simulink model "Calculate_Average_Switching_Frequency"  (R2018a)
settings: Solver=FixedStepAuto  StartTime=0.0  StopTime=0.17  RelTol=1e-3
values from neighbouring files (symbols this model uses):
  f_f_cf = 100e3    (= 100000)    [Init_Average_Switching_Frequency.m]
  f_T_cf = 1/f_f_cf    (= 1e-05)    [Init_Average_Switching_Frequency.m]
  f_T_fpga = 1/f_fpga    (= 1e-08)    [Init_Average_Switching_Frequency.m]
  T_fpga = 1/f_fpga    (= 1e-08)    [Init_Average_Switching_Frequency.m]
undefined symbols (not defined in the file or in its folder): pe
libraries: pe_lib x2, elec_lib x1
settings Model: Creator=Maximlian  LastModifiedBy=Wendel
settings OptimizationCC: BlockReduction=off  ConditionallyExecuteInputs=off  DefaultParameterBehavior=Inlined  EnhancedBackFolding=on  PassReuseOutputArgsAs=Individual arguments  OptimizeBlockOrder=speed  DifferentSizesBufferReuse=on  OptimizationCustomize=off
settings DebuggingCC: AlgebraicLoopMsg=error  ParameterTunabilityLossMsg=error
settings HardwareCC: ProdBitPerPointer=32  ProdBitPerSizeT=32  ProdBitPerPtrDiffT=32  ProdLargestAtomicFloat=None  ProdIntDivRoundTo=Undefined  ProdEndianess=Unspecified  ProdWordSize=32  ProdHWDeviceType=ASIC/FPGA->ASIC/FPGA  TargetBitPerPointer=64  TargetBitPerSizeT=64  TargetBitPerPtrDiffT=64  TargetLongLongMode=on  TargetIntDivRoundTo=Zero  TargetEndianess=LittleEndian  TargetWordSize=64  TargetHWDeviceType=Custom Processor->MATLAB Host Computer  ProdEqTarget=off
settings SFSimCC: MATLABDynamicMemAlloc=off
settings RTWCC: SystemTargetFile=ert.tlc  GenCodeOnly=on  TemplateMakefile=ert_default_tmf  GenerateReport=on  IncludeHyperlinkInReport=on  LaunchReport=on  GenerateTraceInfo=on  GenerateTraceReport=on  GenerateTraceReportSl=on  GenerateTraceReportSf=on  GenerateTraceReportEml=on
settings CodeAppCC: ForceParamTrailComments=on  IgnoreCustomStorageClasses=off  OperatorAnnotations=on  SimulinkDataObjDesc=on  SFDataObjDesc=on  InsertBlockDesc=on
settings ERTTargetCC: TargetLangStandard=C99 (ISO)  GenerateSampleERTMain=on  MultiInstanceERTCode=on  CodeInterfacePackaging=Reusable function  InlinedParameterPlacement=NonHierarchical  ERTCustomFileTemplate=example_file_process.tlc

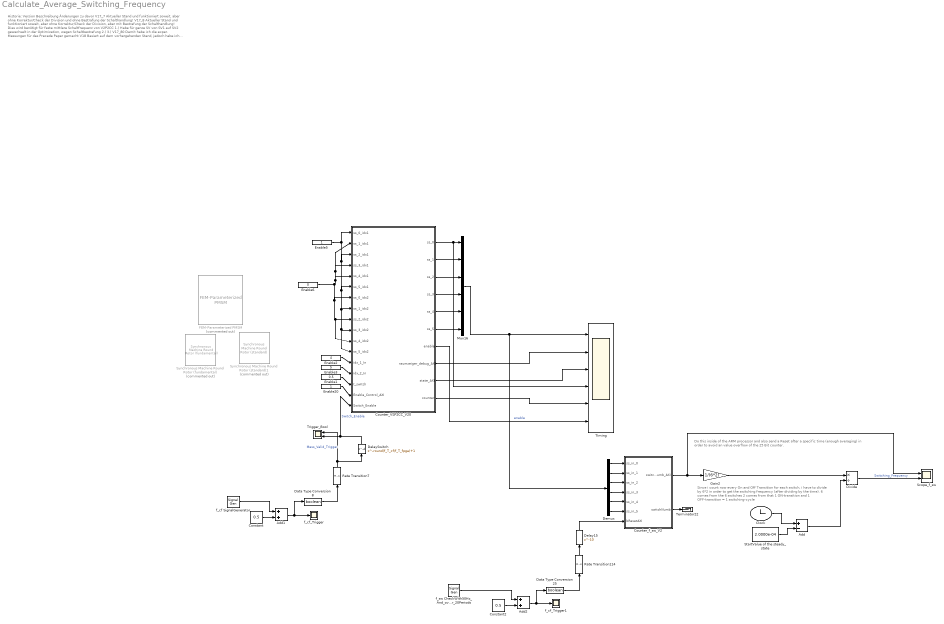
== system Calculate_Average_Switching_Frequency ==
  note: Historie:
      |
      | Version
      | Beschreibung
      | Änderungen zu davor
      |
      | V17_7
      | Aktueller Stand und funktioniert soweit, aber ohne Korrektur/Check der Division und ohne Bestrafung der Schalthandlung!
      |
      | V17_8
      | Aktueller Stand und funktioniert soweit, aber ohne Korrektur/Check der Division, aber mit Bestrafung der Schalthandlung! Dies wird benötigt für feste mittlere Schaltfrequenz von V2P2CC
      | 1.) Habe für ganze SV von SV1 auf SV2 gewechselt in der Optimization, wegen Schaltbestrafung
      | 2.)
      | 3.)
      |
      | V17_80
      | Damit habe ich die exper. Messungen für das Precede Paper gemacht
      |
      | V18
      | Basiert auf dem vorhergehenden Stand, jedoch habe ich hier in Simulation die Scopes angepasst, für gute Plots für das Precede Paper in Simulation
  note: Since i count now every On and Off Transition for each switch,
      |  i have to divide by 6*2 in order to get the switching frequency
      |  (after dividing by the time).
      | 6 comes from the 6 switches
      | 2 comes from that 1 ON-transition and 1 OFF-transition = 1 switching-cycle
  note: Do this inside of the ARM processor and also send a Reset after a specific
      | time (enough averaging) in order to avoid an value overflow of the 25 Bit
      | counter.
  Add : Sum  Inputs=+-
  Add1 : Sum
  Add2 : Sum
  Clock : Clock
  Constant : Constant  Value=0.5
  Constant2 : Constant  Value=0.5
  Counter_VSP2CC_V20 : Subsystem  TreatAsAtomicUnit=on
      mask Display: image('ELSYS_embedded.png');
  Counter_f_sw_V2 : Subsystem  TreatAsAtomicUnit=on
      mask Display: image('ELSYS_embedded.png');
  Data Type Conversion25 : DataTypeConversion  OutDataTypeStr=boolean
  Data Type Conversion8 : DataTypeConversion  OutDataTypeStr=boolean
  Delay15 : Delay  DelayLength=10  InitialCondition=0
  DelaySwitch : Delay  DelayLength=round(f_T_cf/f_T_fpga)+1
  Demux : Demux  Outputs=6
  Divide : Product  Inputs=*/  SaturateOnIntegerOverflow=on  RndMeth=Zero
  Enable1 : Constant  Value=0.5  OutDataTypeStr=fixdt(1,16,11)  SampleTime=T_fpga
  Enable2 : Constant  Value=4  OutDataTypeStr=fixdt(0,4,0)  SampleTime=T_fpga
  Enable20 : Constant  OutDataTypeStr=boolean  SampleTime=T_fpga
  Enable3 : Constant  Value=5  OutDataTypeStr=fixdt(0,4,0)  SampleTime=T_fpga
  Enable5 : Constant  OutDataTypeStr=fixdt(0,1,0)  SampleTime=T_fpga
  Enable6 : Constant  Value=0  OutDataTypeStr=fixdt(0,1,0)  SampleTime=T_fpga
  FEM-Parameterized PMSM : elec_lib/Actuators & Drivers/Rotational Actuators/FEM-Parameterized PMSM  Commented=on  parameterization=1  iVec=[-2, 0, 2] A  xVec=[0, 20, 40, 60] deg  dfluxdiMatrix=0.0002 * ones(3, 4) Wb/A  dfluxdxMatrix=[0, -.16, .16, 0; 0, -.16, .16, 0; 0, -.16, .16, 0] Wb/rad  calculate_torque_matrix=1  TorqueMatrix=zeros(3, 3, 3, 4) N*m  idVec1=[-200, 0, 200] A  iqVec1=[-200, 0, 200] A  LdMatrix=0.0002 * ones(3, 3) H  LqMatrix=0.0002 * ones(3, 3) H  PmMatrix=0.1 * ones(3, 3) Wb  N=6  interp_method=simscape.enum.interpolation.linear  Rs=0.013 Ohm  Ms=0.00002 H  losses_oc=[0, 0, 0] W  losses_sc=[0, 0, 0] W  f_losses=60 Hz  Isc_losses=95 A  Inertia=0.01 kg*m^2  lam=0 N*m/(rad/s)  i_d_specify=off  i_d_priority=None  i_d=0 A  i_d_nominal_specify=off  i_d_nominal_unit=A  i_d_nominal_value=1  i_q_specify=off  i_q_priority=None  i_q=0 A  i_q_nominal_specify=off  i_q_nominal_unit=A  i_q_nominal_value=1  torque_specify=off  torque_priority=None  torque=0 N*m  torque_nominal_specify=off  torque_nominal_unit=N*m  torque_nominal_value=1  angular_velocity_specify=off  angular_velocity_priority=High  angular_velocity=0 rpm  angular_velocity_nominal_specify=off  angular_velocity_nominal_unit=rpm  angular_velocity_nominal_value=1  angular_position_specify=off  angular_position_priority=High  angular_position=0 deg  angular_position_nominal_specify=off  angular_position_nominal_unit=deg  angular_position_nominal_value=1  Tmeas=298.15 K  alpha=3.93e-3 1/K  alpha_flux=-0.001 1/K  stator_thermal_mass=100 J/K  stator_initial_temperatures=[298.15, 298.15, 298.15] K  rotor_thermal_mass=200 J/K  rotor_initial_temperature=298.15 K  Rm_percent_rotor=90  Rd_percent_rotor=30  idVec=[-200, 0, 200] A  iqVec=[-200, 0, 200] A  dfluxAdiaMatrix3D=zeros(3, 3, 4) Wb/A  dfluxAdibMatrix3D=zeros(3, 3, 4) Wb/A  dfluxAdicMatrix3D=zeros(3, 3, 4) Wb/A  dfluxAdxMatrix3D=zeros(3, 3, 4) Wb/rad  TorqueMatrix3D=zeros(3, 3, 4) N*m  iaVec=[-200, 0, 200] A  ibVec=[-200, 0, 200] A  icVec=[-200, 0, 200] A  dfluxAdiaMatrix=zeros(3, 3, 3, 4) Wb/A  dfluxAdibMatrix=zeros(3, 3, 3, 4) Wb/A  dfluxAdicMatrix=zeros(3, 3, 3, 4) Wb/A  dfluxAdxMatrix=zeros(3, 3, 3, 4) Wb/rad  winding_type_dq0=1  nPolePairs=4  parks_type=1  idVec2=[-200, 0, 200] A  iqVec2=[-200, 0, 200] A  xVec2=[0, 10, 20, 30] deg  fluxD_dq0=zeros(3, 3, 4) Wb  fluxQ_dq0=zeros(3, 3, 4) Wb  Torque_dq0=zeros(3, 3, 4) N*m
      settings: SourceProductName=Simscape Electronics  SourceProductBaseCode=SN
  Gain2 : Gain  Gain=1/(6*2)
  Mux16 : Mux  Inputs=6
  Rate Transition114 : RateTransition  OutPortSampleTime=T_fpga
  Rate Transition7 : RateTransition  OutPortSampleTime=T_fpga
  Scope_f_sw : Scope  NumInputPorts=2
  StartValue of the steady_state : Constant  Value=2.0000e-04  SampleTime=-1
  Synchronous Machine Round Rotor (fundamental) : pe_lib/Machines/Synchronous Machine (Round Rotor)/Synchronous Machine Round Rotor (fundamental)  Commented=on  SRated=555e6 V*A  VRated=24e3 V  FRated=60 Hz  nPolePairs=1  fieldCircuitParameterization_option=2  baseEfd=92.95 V  baseIfd=1300 A  zero_sequence=pe.enum.park.zerosequence.include  Ladu=1.66  Laqu=1.61  L0=0.15  Ll=0.15  Ra=0.003  Lfd=0.165  Rfd=0.0006  L1d=0.1713  R1d=0.0284  L1q=0.7252  R1q=0.00619  L2q=0.125  R2q=0.02368  saturation_option=0  saturation_ifd=[0, .48, .76, 1.38, 1.79]  saturation_Vag=[0, .8, 1.08, 1.31, 1.4]  initialization_option=2  angular_position0=0 deg  pu_psid0=0  pu_psiq0=0  pu_psi00=0  pu_psifd0=0  pu_psi1d0=0  pu_psi1q0=0  pu_psi2q0=0  Vmag0=24e3 V  Vang0=0 deg  Pt0=500e6 V*A  Qt0=0 V*A  shift_3ph=[nan, nan, nan] rad  connection_option=int32(pe.Connection.wye)  num_q_dampers=2  oneOverOmega=nan s/rad  Lmin=1e-9  base_v=nan V  base_i=nan A  base_torque=nan N*m  base_wMechanical=nan rad/s  base_rc_efd=nan V  base_rc_ifd=nan A  base_fd_Efd=nan V  base_fd_Ifd=nan A  saturation_psi=0  saturation_K_s=1
      settings: SourceProductName=Simscape Power Systems  SourceProductBaseCode=PS
  Synchronous Machine Round Rotor (standard)1 : pe_lib/Machines/Synchronous Machine (Round Rotor)/Synchronous Machine Round Rotor (standard)  Commented=on  SRated=555e6 V*A  VRated=24e3 V  FRated=60 Hz  nPolePairs=1  fieldCircuitParameterization_option=1  baseEfd=92.95 V  baseIfd=1300 A  zero_sequence=pe.enum.park.zerosequence.include  Ra=0.003  Xl=0.15  Xd=1.81  Xq=1.76  X0=0.15  Xdd=0.3  Xqd=0.65  Xddd=0.23  Xqdd=0.25  d_transient_option=1  Td0d=8 s  Tdd=1.3260 s  d_subtransient_option=1  Td0dd=0.03 s  Tddd=0.0230 s  q_transient_option=1  Tq0d=1 s  Tqd=0.3693 s  q_subtransient_option=1  Tq0dd=0.07 s  Tqdd=0.0269 s  saturation_option=1  saturation_ifd=[0, .48, .76, 1.38, 1.79]  saturation_Vag=[0, .8, 1.08, 1.31, 1.4]  initialization_option=2  angular_position0=0 deg  pu_psid0=0  pu_psiq0=0  pu_psi00=0  pu_psifd0=0  pu_psi1d0=0  pu_psi1q0=0  pu_psi2q0=0  Vmag0=24e3 V  Vang0=0 deg  Pt0=500e6 V*A  Qt0=0 V*A  shift_3ph=[nan, nan, nan] rad  connection_option=int32(pe.Connection.wye)  num_q_dampers=2  oneOverOmega=nan s/rad  L0=nan  Ladu=nan  Laqu=nan  Ll=nan  Lfd=nan  Rfd=nan  L1d=nan  R1d=nan  L1q=nan  R1q=nan  L2q=nan  R2q=nan  Xmin=1e-9  base_v=nan V  base_i=nan A  base_torque=nan N*m  base_wMechanical=nan rad/s  base_rc_efd=nan V  base_rc_ifd=nan A  base_fd_Efd=nan V  base_fd_Ifd=nan A  saturation_psi=0  saturation_K_s=1
      settings: SourceProductName=Simscape Power Systems  SourceProductBaseCode=PS
  Terminator22 : Terminator
  Timing : Scope  NumInputPorts=6
  Trigger_Bool : Scope  NumInputPorts=2
  f_cf SignalGenerator : SignalGenerator  WaveForm=square  Amplitude=0.5  Frequency=f_f_cf
  f_cf_Trigger : Scope
  f_cf_Trigger1 : Scope
  f_sw CheckWith50Hz_And_over_20Periods : SignalGenerator  WaveForm=square  Amplitude=0.5  Frequency=50
  wires:
  Counter_VSP2CC_V20/10(counter) -> Timing/5
  Counter_VSP2CC_V20/1(ss_0) -> Timing/4, Mux16/1
  Counter_VSP2CC_V20/3(ss_2) -> Mux16/3
  Counter_VSP2CC_V20/4(ss_3) -> Mux16/4
  Counter_VSP2CC_V20/6(ss_5) -> Mux16/6
  Counter_VSP2CC_V20/7(enable) -> Timing/6  "enable"
  Counter_VSP2CC_V20/2(ss_1) -> Mux16/2
  Counter_VSP2CC_V20/5(ss_4) -> Mux16/5
  Enable20/1 -> Counter_VSP2CC_V20/16(Enable_Control_AXI)
  Enable1/1 -> Counter_VSP2CC_V20/15(t_switch)
  Enable3/1 -> Counter_VSP2CC_V20/14(idx_2_In)
  Enable2/1 -> Counter_VSP2CC_V20/13(idx_1_In)
  Enable5/1 -> Counter_VSP2CC_V20/8(ss_1_idx2), Counter_VSP2CC_V20/10(ss_3_idx2), Counter_VSP2CC_V20/12(ss_5_idx2), Counter_VSP2CC_V20/6(ss_5_idx1), Counter_VSP2CC_V20/3(ss_2_idx1), Counter_VSP2CC_V20/1(ss_0_idx1)
  Enable6/1 -> Counter_VSP2CC_V20/11(ss_4_idx2), Counter_VSP2CC_V20/9(ss_2_idx2), Counter_VSP2CC_V20/7(ss_0_idx2), Counter_VSP2CC_V20/5(ss_4_idx1), Counter_VSP2CC_V20/4(ss_3_idx1), Counter_VSP2CC_V20/2(ss_1_idx1)
  Counter_VSP2CC_V20/8(raumzeiger_debug_AXI) -> Timing/2
  Counter_VSP2CC_V20/9(state_AXI) -> Timing/3
  Data Type Conversion8/1 -> Rate Transition7/1
  Constant/1 -> Add1/2
  Rate Transition7/1 -> Trigger_Bool/1, DelaySwitch/1  "Mess_Valid_Trigger"
  Add1/1 -> Data Type Conversion8/1, f_cf_Trigger/1
  f_cf SignalGenerator/1 -> Add1/1
  DelaySwitch/1 -> Counter_VSP2CC_V20/17(Switch_Enable), Trigger_Bool/2  "Switch_Enable"
  Counter_f_sw_V2/1(switchNumb_AXI) -> Gain2/1, Scope_f_sw/1
  Clock/1 -> Add/1
  Add2/1 -> Data Type Conversion25/1, f_cf_Trigger1/1
  StartValue of the steady_state/1 -> Add/2
  Demux/3 -> Counter_f_sw_V2/3(ss_in_2)
  Demux/5 -> Counter_f_sw_V2/5(ss_in_4)
  Rate Transition114/1 -> Delay15/1
  Demux/1 -> Counter_f_sw_V2/1(ss_in_0)
  Demux/6 -> Counter_f_sw_V2/6(ss_in_5)
  Delay15/1 -> Counter_f_sw_V2/7(bResetAXI)
  Gain2/1 -> Divide/1
  Data Type Conversion25/1 -> Rate Transition114/1
  Divide/1 -> Scope_f_sw/2  "Switching_Frequency"
  Add/1 -> Divide/2
  f_sw CheckWith50Hz_And_over_20Periods/1 -> Add2/1
  Constant2/1 -> Add2/2
  Counter_f_sw_V2/2(switchNumb) -> Terminator22/1
  Demux/2 -> Counter_f_sw_V2/2(ss_in_1)
  Demux/4 -> Counter_f_sw_V2/4(ss_in_3)
  Mux16/1 -> Demux/1, Timing/1

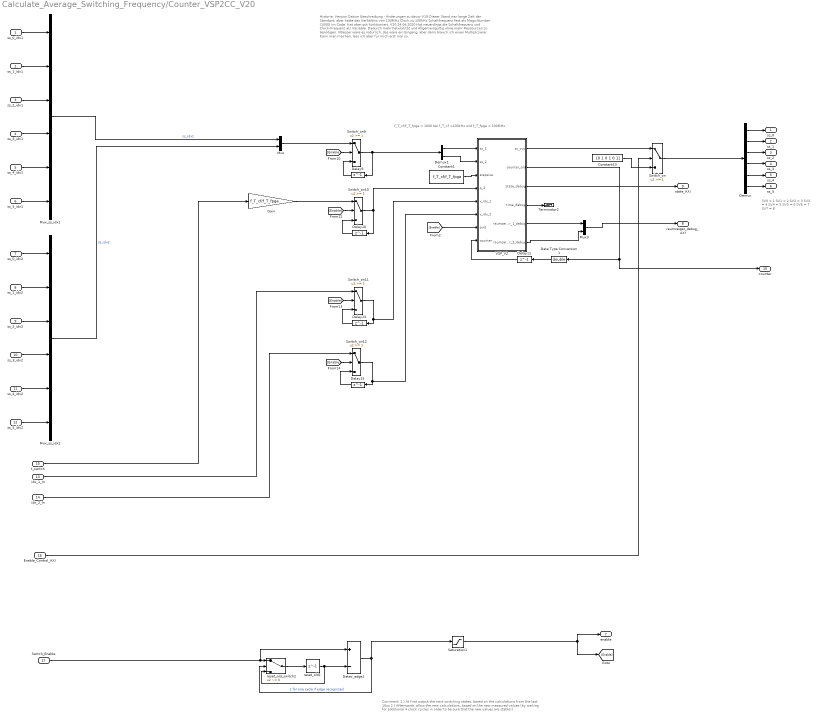
== system Calculate_Average_Switching_Frequency/Counter_VSP2CC_V20 ==
  note: Comment:
      | 1.) At first output the next switching states, based on the calculations from the last 10us
      | 2.) Afterwards, allow the new calculations, based on the new measured values
      | (by waiting for additional 4 clock cycles in order to be sure that the new values are stable!)
  note: SV0 = 1
      | SV1 = 2
      | SV2 = 3
      | SV3 = 4
      | SV4 = 5
      | SV5 = 6
      | SV6 = 7
      | SV7 = 8
  note: f_T_cf/f_T_fpga = 1000 bei f_T_cf =100kHz und f_T_fpga = 100MHz
  note: Historie:
      |
      | Version
      | Datum
      | Beschreibung - Änderungen zu davor
      |
      | V19
      |
      | Dieser Stand war lange Zeit der Standard, aber hatte das Verhältnis von 100MHz Clock zu 100kHz Schaltfrequenz fest als MagicNumber (1000) im Code. Hat aber gut funktioniert.
      |
      | V20
      | 24.04.2020
      | Hat neuerdings die Schaltfrequenz und Clock-Frequenz als Variable. Dadurch mehr Felxibilität und Allgemeingültig ohne mehr Ressourcen zu benötigen.
      | VBesser wäre es natürlich, das wäre ein Eingang, aber dann brauch ich einen Multiplizierer. Kann man machen, lass ich aber für mich erst mal so.
  ss_0_idx1 : Inport
  ss_1_idx1 : Inport  Port=2
  ss_2_idx1 : Inport  Port=3
  ss_3_idx1 : Inport  Port=4
  ss_4_idx1 : Inport  Port=5
  ss_5_idx1 : Inport  Port=6
  ss_0_idx2 : Inport  Port=7
  ss_1_idx2 : Inport  Port=8
  ss_2_idx2 : Inport  Port=9
  ss_3_idx2 : Inport  Port=10
  ss_4_idx2 : Inport  Port=11
  ss_5_idx2 : Inport  Port=12
  idx_1_In : Inport  Port=13
  idx_2_In : Inport  Port=14
  t_switch : Inport  Port=15
  Enable_Control_AXI : Inport  Port=16
  Switch_Enable : Inport  Port=17
  Constant1 : Constant  Value=f_T_cf/f_T_fpga  OutDataTypeStr=double  SampleTime=f_T_fpga
  Constant13 : Constant  Value=[0 1 0 1 0 1]  OutDataTypeStr=boolean  SampleTime=f_T_fpga
  Data Type Conversion1 : DataTypeConversion  OutDataTypeStr=double
  Delay{9..11,13,15} (5 alike) : Delay  DelayLength=1
  Demux : Demux  Outputs=6
  Demux1 : Demux  Outputs=2
  Detec_edge1 : Sum  Inputs=+-  AccumDataTypeStr=int8  OutDataTypeStr=int8
  Gain : Gain  Gain=f_T_cf/f_T_fpga
  Mux : Mux  Inputs=2
  Mux3 : Mux  Inputs=2
  Mux_ss_idx1 : Mux  Inputs=6
  Mux_ss_idx2 : Mux  Inputs=6
  Saturation1 : Saturate  UpperLimit=1  LowerLimit=0  OutMin=[0]  OutMax=[1]  OutDataTypeStr=fixdt(0,1)
  Switch_on : Switch  Threshold=1
  Switch_on10 : Switch  Threshold=1  OutDataTypeStr=double
  Switch_on11 : Switch  Threshold=1  OutDataTypeStr=fixdt(0,4,0)
  Switch_on12 : Switch  Threshold=1  OutDataTypeStr=fixdt(0,4,0)
  Switch_on9 : Switch  Threshold=1  OutDataTypeStr=fixdt(0,1,0)
  Terminator2 : Terminator
  VSP_V2 : MATLAB Function  TreatAsAtomicUnit=on
  reset_old1 : Delay  DelayLength=1
  reset_old_switch2 : Switch  Criteria=u2 ~= 0
  ss_0 : Outport
  ss_1 : Outport  Port=2
  ss_2 : Outport  Port=3
  ss_3 : Outport  Port=4
  ss_4 : Outport  Port=5
  ss_5 : Outport  Port=6
  enable : Outport  Port=7
  raumzeiger_debug_AXI : Outport  Port=8
  state_AXI : Outport  Port=9
  counter : Outport  Port=10
  wires:
  Saturation1/1 -> [Enable], enable/1
  VSP_V2/1(ss_out) -> Switch_on/1
  VSP_V2/2(counter_old) -> counter/1, Data Type Conversion1/1
  VSP_V2/3(state_debug) -> state_AXI/1
  [Enable] -> VSP_V2/7(puls)
  Demux1/1 -> VSP_V2/1(ss_1)
  Demux1/2 -> VSP_V2/2(ss_2)
  [Enable] -> Switch_on10/2
  Delay10/1 -> Switch_on10/3
  [Enable] -> Switch_on9/2
  Switch_on9/1 -> Demux1/1, Delay9/1
  Delay9/1 -> Switch_on9/3
  VSP_V2/5(raumzeiger_1_debug) -> Mux3/1
  VSP_V2/6(raumzeiger_2_debug) -> Mux3/2
  Mux3/1 -> raumzeiger_debug_AXI/1
  Switch_on10/1 -> Delay10/1, VSP_V2/4(p_2)
  [Enable] -> Switch_on11/2
  Switch_on11/1 -> VSP_V2/5(v_idx_1), Delay13/1
  Delay13/1 -> Switch_on11/3
  idx_1_In/1 -> Switch_on11/1
  Delay15/1 -> Switch_on12/3
  [Enable] -> Switch_on12/2
  Switch_on12/1 -> VSP_V2/6(v_idx_2), Delay15/1
  idx_2_In/1 -> Switch_on12/1
  Mux/1 -> Switch_on9/1
  Detec_edge1/1 -> Saturation1/1, reset_old_switch2/2  "1 for one cycle if edge recognized"
  reset_old1/1 -> reset_old_switch2/3, Detec_edge1/2
  reset_old_switch2/1 -> reset_old1/1
  Switch_Enable/1 -> Detec_edge1/1, reset_old_switch2/1
  Constant1/1 -> VSP_V2/3(stepsize)
  Data Type Conversion1/1 -> Delay11/1
  Delay11/1 -> VSP_V2/8(counter)
  VSP_V2/4(time_debug) -> Terminator2/1
  t_switch/1 -> Gain/1
  Demux/3 -> ss_2/1
  Demux/2 -> ss_1/1
  Demux/5 -> ss_4/1
  Demux/4 -> ss_3/1
  Demux/6 -> ss_5/1
  Demux/1 -> ss_0/1
  Enable_Control_AXI/1 -> Switch_on/2
  Constant13/1 -> Switch_on/3
  Switch_on/1 -> Demux/1
  Mux_ss_idx1/1 -> Mux/1  "ss_idx1"
  ss_5_idx1/1 -> Mux_ss_idx1/6
  ss_4_idx1/1 -> Mux_ss_idx1/5
  ss_3_idx1/1 -> Mux_ss_idx1/4
  ss_2_idx1/1 -> Mux_ss_idx1/3
  ss_0_idx1/1 -> Mux_ss_idx1/1
  ss_1_idx1/1 -> Mux_ss_idx1/2
  ss_2_idx2/1 -> Mux_ss_idx2/3
  ss_1_idx2/1 -> Mux_ss_idx2/2
  ss_0_idx2/1 -> Mux_ss_idx2/1
  ss_3_idx2/1 -> Mux_ss_idx2/4
  ss_5_idx2/1 -> Mux_ss_idx2/6
  Mux_ss_idx2/1 -> Mux/2  "ss_idx2"
  ss_4_idx2/1 -> Mux_ss_idx2/5
  Gain/1 -> Switch_on10/1

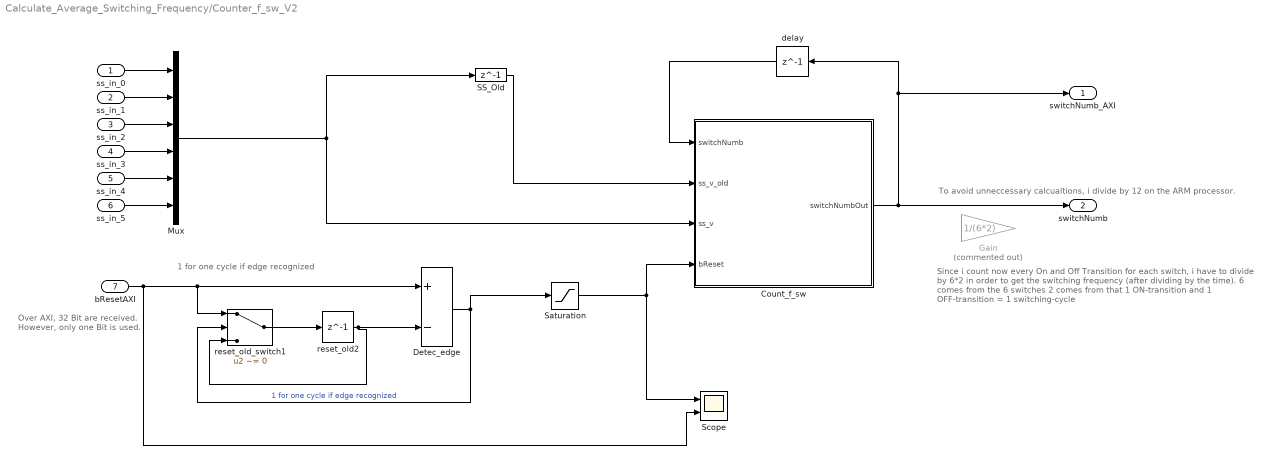
== system Calculate_Average_Switching_Frequency/Counter_f_sw_V2 ==
  note: To avoid unneccessary calcualtions, i divide by 12 on the ARM processor.
  note: Over AXI, 32 Bit are received.
      | However, only one Bit is used.
  note: 1 for one cycle if edge recognized
  note: Since i count now every On and Off Transition for each switch,
      |  i have to divide by 6*2 in order to get the switching frequency
      |  (after dividing by the time).
      | 6 comes from the 6 switches
      | 2 comes from that 1 ON-transition and 1 OFF-transition = 1 switching-cycle
  ss_in_0 : Inport
  ss_in_1 : Inport  Port=2
  ss_in_2 : Inport  Port=3
  ss_in_3 : Inport  Port=4
  ss_in_4 : Inport  Port=5
  ss_in_5 : Inport  Port=6
  bResetAXI : Inport  Port=7
  Count_f_sw : MATLAB Function  TreatAsAtomicUnit=on  VariantControl=(default)
  Detec_edge : Sum  Inputs=+-  AccumDataTypeStr=int8  OutDataTypeStr=int8
  Gain : Gain  Commented=on  Gain=1/(6*2)
  Mux : Mux  Inputs=6
  SS_Old : Delay  DelayLength=1
  Saturation : Saturate  UpperLimit=1  LowerLimit=0  OutMin=[0]  OutMax=[1]  OutDataTypeStr=fixdt(0,1)
  Scope : Scope  NumInputPorts=2
  delay : Delay  DelayLength=1
  reset_old2 : Delay  DelayLength=1
  reset_old_switch1 : Switch  Criteria=u2 ~= 0
  switchNumb_AXI : Outport
  switchNumb : Outport  Port=2
  wires:
  Saturation/1 -> Count_f_sw/4(bReset), Scope/1
  Count_f_sw/1(switchNumbOut) -> delay/1, switchNumb_AXI/1, switchNumb/1
  reset_old_switch1/1 -> reset_old2/1
  bResetAXI/1 -> Scope/2, reset_old_switch1/1, Detec_edge/1
  reset_old2/1 -> Detec_edge/2, reset_old_switch1/3
  Detec_edge/1 -> Saturation/1, reset_old_switch1/2  "1 for one cycle if edge recognized"
  delay/1 -> Count_f_sw/1(switchNumb)
  ss_in_0/1 -> Mux/1
  ss_in_5/1 -> Mux/6
  ss_in_4/1 -> Mux/5
  ss_in_3/1 -> Mux/4
  ss_in_2/1 -> Mux/3
  ss_in_1/1 -> Mux/2
  Mux/1 -> Count_f_sw/3(ss_v), SS_Old/1
  SS_Old/1 -> Count_f_sw/2(ss_v_old)

== matlab function Calculate_Average_Switching_Frequency/Counter_VSP2CC_V20/VSP_V2 ==
  data: ss_1 input; ss_out output; ss_2 input; stepsize input; p_2 input; v_idx_1 input; v_idx_2 input; counter_old output; state_debug output; time_debug output; raumzeiger_1_debug output; puls input; raumzeiger_2_debug output; counter input
function [ss_out,counter_old,state_debug,time_debug,raumzeiger_1_debug,raumzeiger_2_debug]   = fcn(ss_1, ss_2,stepsize,p_2,v_idx_1,v_idx_2,puls, counter)
    
 Fq16    = fimath('RoundingMethod', 'Floor', 'OverflowAction', 'Wrap','ProductMode', 'FullPrecision', 'ProductWordLength', 16,'ProductFractionLength',0,'SumMode','SpecifyPrecision','SumWordLength',16,'SumFractionLength',0);

%    persistent counter;
    if isempty(counter)
        counter = 0; 
    end

    ss_temp = fi([0;
              1;
              0;
              1;
              0;
              1;
              ],0,1,0);
    
    if puls == 1
        counter = 0;
    end
    
    counter= counter+1;
    
    if counter > stepsize
        counter = stepsize;
    end
    
    state_temp = fi(0, 0, 4, 0);
    v_temp_1 = fi(v_idx_1, 0, 4, 0); % Selected space vector 1
    v_temp_2 = fi(v_idx_2, 0, 4, 0); % Selected space vector 1
    
    if counter<=(p_2)
        ss_temp = fi(ss_1,0,1,0);
        state_temp = fi(1, 0, 4, 0);
        %v_temp_1=v_idx_1;
        
    elseif (counter > p_2)
        ss_temp = fi(ss_2,0,1,0);
        state_temp = fi(2, 0, 4, 0);
        %v_temp_2=v_idx_2;
    else %This state should be never reached (outputs zero SV)
        ss_temp = fi([0;
                      1;
                      0;
                      1;
                      0;
                      1;
                      ],0,1,0);
    end
     
    ss_out=[ss_temp(1);
        ss_temp(2);
        ss_temp(3);
        ss_temp(4);
        ss_temp(5);
        ss_temp(6);
        ];
    
    counter_old = counter;
    state_debug=state_temp;
    time_debug=p_2;
    raumzeiger_1_debug=v_temp_1;
    raumzeiger_2_debug=v_temp_2;  

end

== matlab function Calculate_Average_Switching_Frequency/Counter_f_sw_V2/Count_f_sw ==
  data: switchNumb input fixdt(0,25,0); ss_v_old input; ss_v input; switchNumbOut output fixdt(0,25,0); bReset input
 function switchNumbOut   = Count_f_sw(switchNumb,ss_v_old,ss_v, bReset)
   %
    %% toDO
        %s
 
    %% Initialization
    Fq25    = fimath('RoundingMethod', 'Floor', 'OverflowAction', 'Wrap','ProductMode', 'FullPrecision', 'ProductWordLength', 25,'ProductFractionLength',0,'SumMode','SpecifyPrecision','SumWordLength',25,'SumFractionLength',0);

    % I need this initialization, in order that the HDL Coder and Simulink knows the size of the vectors! Without these, i will get an error!
   % idx_globalOld     = fi(1, 0, 8, 0); % Chosen position overall in the error vector
    %switchNumb = fi(0, 0, 25, 0);
    
    %% Reset the counters (similar to the THD, i will try to average the switching frequency over 20 fundamental periods. After this time, a Reset-Flag from the ARM processor will reset the counter) 
    if (bReset == true) 
        switchNumb = fi(0, 0, 25, 0);
    end
    %% Check if switching occurs. If yes count up.
    % However, dependent of the ss_v before, switching can but do not have to occure, if the previously applied ss_v keeps.

    %Use a for-loop since in VHDL i have time and can do a resource streaming
    %Even if i need 6 cycles @100MHz, since it is not able to have have
    %switching (on/off inside of 60ns), this is ok (because T_cf = 10us and
    %and switching for such a short time is not allwoed nayway, since it is
    %not worth it (too much losses).)
    for countSS=fi(1, 0, 8, 0):fi(6, 0, 8, 0) %1:6
        if (ss_v(countSS) ~= ss_v_old(countSS)) %Check if switch has changed
            switchNumb = fi(add(Fq25,switchNumb,fi(1, 0, 25, 0)),0,25,0); % +1 Increment the switch counter +1
        end
    end

    switchNumbOut = switchNumb;

 end
